simulink model "npc_controller"  (R2022a)
settings: Solver=FixedStepDiscrete  StartTime=0.0  StopTime=20  RelTol=1e-3  EnableMultiTasking=on
values from neighbouring files (symbols this model uses):
  Tsw = 1.5E-5    [param.sldd]
undefined symbols (not defined in the file or in its folder): CAN_O_INT, CANA_BASE, Down, GPTRIP1SEL, GPTRIP2SEL, GPTRIP3SEL, TZ1, TZ2, TZ3, Up
libraries: simulink x153, hdlsllib x90, c2802xlib x34, c2837xDlib x18, c280xlib x12, canmsglib x9, c2838xlib x8, idelinklib_common x3, c2806xlib x2, slpidlib x2, c28004xlib x2, c281xlib x2
(part 42 of 45)

== system npc_controller/IDLE_AND_TIMER/codegen/CAN_Task/Tx_Handler/Run Tx Routine/TxStatusData/Tx Pri3 ID132/Float Data to Bytes3 ==
  Float Data : Inport
  Resol. : Inport  Port=2
  Bit Shift : hdlsllib/Logic and Bit Operations/Bit Shift  mode=Shift Right Logical  N=8
  Bitwise AND : simulink/Logic and Bit Operations/Bitwise Operator  logicop=AND  UseBitMask=on  BitMask=bin2dec('0000000011111111')  BitMaskRealWorld=Stored Integer
  Bitwise AND1 : simulink/Logic and Bit Operations/Bitwise Operator  logicop=AND  UseBitMask=on  BitMask=hex2dec('FF00')  BitMaskRealWorld=Stored Integer
  Data Type Conversion : DataTypeConversion  OutDataTypeStr=uint8  SaturateOnIntegerOverflow=off  RndMeth=Floor
  Data Type Conversion1 : DataTypeConversion  OutDataTypeStr=uint8  SaturateOnIntegerOverflow=off  RndMeth=Floor
  Data Type Conversion2 : DataTypeConversion  OutDataTypeStr=uint16  SaturateOnIntegerOverflow=off  RndMeth=Floor
  Divide : Product  Inputs=*/
  u8Lsb : Outport
  u8Msb : Outport  Port=2
  wires:
  Data Type Conversion/1 -> u8Lsb/1
  Bitwise AND1/1 -> Bit Shift/1
  Data Type Conversion1/1 -> u8Msb/1
  Bitwise AND/1 -> Data Type Conversion/1
  Bit Shift/1 -> Data Type Conversion1/1
  Data Type Conversion2/1 -> Bitwise AND1/1, Bitwise AND/1  "u16toBytes_1"
  Divide/1 -> Data Type Conversion2/1
  Float Data/1 -> Divide/1
  Resol./1 -> Divide/2

== stateflow chart npc_controller/IDLE_AND_TIMER/codegen/Chart1 ==
  state INIT
    en:
    sim_control;
  (default) -> INIT
  INIT -> INIT
  events: sim_control output FUNCTION_CALL_EVENT

== stateflow chart npc_controller/CONTROL/STATE-MACHINE/CPU_CONTROL_200_Vpk ==
  state configGrid(grid_config,   sinlgeph_config) [function] [commented out]
  state enDigCmpMode [function]
  state configFutEn [function]
  state disDigCmpMode [function]
  state configFutDis [function]
  state theta = updatePll3p(van, vbn, vcn) [function] [commented out]
  state calib_ok = updateCalib(cnt_calib, van, vbn, vcn, ia, ib, ic) [function]
  state disablePwm [function]
  state tfv_v_UvpOvp = detectUvpOvp(Vpk) [function]
  state phx_en = detectZCPhA(vxn) [function]
  state phx_en = detectZCPhB(vxn) [function]
  state phx_en = detectZCPhC(vxn) [function]
  state vx_seq = updateSequencePhA(vxn, ix) [function]
  state vx_seq = updateSequencePhB(vxn, ix) [function]
  state vx_seq = updateSequencePhC(vxn, ix) [function]
  (default) -> (junction 597)
  (junction 598) -> (junction 531) [order 1] : [calib_ok]
  (junction 597) -> (junction 598) [order 1] : [start_cnt>33333] //50cycles
  (junction 531) -> (junction 14)
  (junction 597) -> (junction 601) [order 2] : {start_cnt++;}
  (junction 598) -> (junction 539) [order 2] : {
      | calib_ok = updateCalib(cnt_calib, van, vbn, vcn, ia, ib, ic);
      | state = 0;
      | }
  (junction 14) -> (junction 542) [order 2]
  (junction 14) -> (junction 128) [order 1] : [tfv_va || tfv_vb || tfv_vc || tfv_iphasea || tfv_iphaseb || tfv_iphasec || tfv_vbulk || tfv_vmid /*|| tfv_vtop*/ || tfv_vaux || tz_ocp || tz_ovp || fault]
      | {
      | fault = true;
      | state = 1;
      | }
  (junction 542) -> (junction 501)
  (junction 501) -> (junction 544) [order 2]
  (junction 501) -> (junction 490) [order 1] : [fut_en_req]
  (junction 544) -> (junction 504)
  (junction 490) -> (junction 492) [order 1] : [!fut_en]
  (junction 504) -> (junction 506) [order 1] : [fut_en]
  (junction 492) -> (junction 498) : {
      | configFutEn();
      | fut_en = true;
      | }
  (junction 490) -> (junction 494) [order 2]
  (junction 504) -> (junction 512) [order 2]
  (junction 506) -> (junction 508) : {
      | configFutDis();
      | fut_en = false;
      | }
  (junction 494) -> (junction 498)
  (junction 508) -> (junction 512)
  (junction 498) -> (junction 520) : {state = 2;}
  (junction 512) -> (junction 346)
  (junction 346) -> (junction 339) [order 1] : [vbulk > 618] //140V
  (junction 346) -> (junction 557) [order 2]
  (junction 339) -> (junction 329) : {
      | control_en = true;
      | enDigCmpMode();
      | }
  (junction 557) -> (junction 560) [order 1] : [vbulk < 530] //120V
  (junction 557) -> (junction 558) [order 2]
  (junction 560) -> (junction 559) : {control_en = false;}
  (junction 558) -> (junction 559)
  (junction 559) -> (junction 329)
  (junction 329) -> (junction 114) [order 1] : [control_en]
  (junction 114) -> (junction 266) [order 1] : [vbulk > 1104] //250V
  (junction 329) -> (junction 580) [order 2]
  (junction 114) -> (junction 263) [order 2]
  (junction 266) -> (junction 273) : {
      | eoss = false;
      | burst_en = true;
      | }
  (junction 263) -> (junction 264) [order 1] : [vbulk < 883] //200V
  (junction 263) -> (junction 267) [order 2]
  (junction 264) -> (junction 270) : {burst_en = false;}
  (junction 267) -> (junction 270)
  (junction 270) -> (junction 273)
  (junction 273) -> (junction 276) [order 1] : [burst_en]
  (junction 273) -> (junction 254) [order 2]
  (junction 276) -> (junction 327) : {
      | disablePwm();
      | va_seq = uint8(0); //forced zero
      | vb_seq = uint8(0);
      | vc_seq = uint8(0);
      | pha_en = false;
      | phb_en = false;
      | phc_en = false;
      | state = 5;
      | }
  (junction 254) -> (junction 606) [order 1] : [eoss]
      | //{tfv_v_UvpOvp = detectUvpOvp(Vpk)}
  (junction 606) -> (junction 256) [order 1] : [1/*!tfv_v_UvpOvp*/]
  (junction 254) -> (junction 97) [order 2]
  (junction 606) -> (junction 607) [order 2]
  (junction 256) -> (junction 101)
  (junction 580) -> (junction 581) [commented out] : [(grid_config_req != grid_config) || (singleph_config_req != singleph_config)]
  (junction 97) -> (junction 93) [order 1] : [(single(883)-vbulk) > single(50)] //11V ripple
  (junction 580) -> (junction 583)
  (junction 581) -> (junction 582) [commented out] : {
      | configGrid(grid_config,   singleph_config);
      | grid_config = grid_config_req;
      | singleph_config = singleph_config_req;
      | }
  (junction 97) -> (junction 110) [order 2]
  (junction 93) -> (junction 109) : {ref = vbulk + single(50);
      | eoss = false;}
  (junction 110) -> (junction 96) [order 1] : [(single(883)-vbulk) < single(-50)]
  (junction 110) -> (junction 94) [order 2] : {ref = single(883); //200V
      | eoss = true;}
  (junction 96) -> (junction 108) : {ref = vbulk - single(50);
      | eoss = false;}
  (junction 101) -> (junction 352) [order 1] : [pha_en]
  (junction 109) -> (junction 101)
  (junction 582) -> (junction 583) [commented out]
  (junction 94) -> (junction 108)
  (junction 108) -> (junction 109)
  (junction 101) -> (junction 356) [order 2] : {
      | va_seq = uint8(0);
      | pha_en = detectZCPhA(van);
      | }
  (junction 352) -> (junction 354) : {va_seq = updateSequencePhA(van, ia);}
  (junction 583) -> (junction 133)
  (junction 356) -> (junction 354)
  (junction 354) -> (junction 362) [order 1] : [phb_en]
  (junction 354) -> (junction 365) [order 2] : {
      | vb_seq = uint8(0);
      | phb_en = detectZCPhB(vbn);
      | }
  (junction 362) -> (junction 366) : {vb_seq = updateSequencePhB(vbn, ib);}
  (junction 365) -> (junction 366)
  (junction 366) -> (junction 367) [order 1] : [phc_en]
  (junction 366) -> (junction 370) [order 2] : {
      | vc_seq = uint8(0);
      | phc_en = detectZCPhC(vcn);
      | }
  (junction 367) -> (junction 372) : {vc_seq = updateSequencePhC(vcn, ic);}
  (junction 370) -> (junction 372)
  (junction 372) -> (junction 299) : {state = 4;}
  (junction 128) -> (junction 133) : //{calib_ok = false;} //calib_ok resets at fault or CAN command
  (junction 133) -> (junction 607)
  (junction 607) -> (junction 299) : {
      | disablePwm();
      | control_en = false;
      | eoss = false;
      | disDigCmpMode();
      | pha_en = false;
      | phb_en = false;
      | phc_en = false;
      | ref = vbulk;
      | state = 3;
      | }
  (junction 299) -> (junction 327)
  (junction 327) -> (junction 533)
  (junction 539) -> (junction 520)
  (junction 520) -> (junction 533)
  (junction 601) -> (junction 539)
  data: grid_config function_input double size=1; sinlgeph_config function_input double size=1; van function_input double size=1; vbn function_input double size=1; vcn function_input double size=1; theta function_output double size=1; calib_ok function_output; cnt_calib function_input uint16 size=1; van function_input single size=1; vbn function_input single size=1; vcn function_input single size=1; ia function_input single size=1; ib function_input single size=1; ic function_input single size=1; Vpk function_input; tfv_v_UvpOvp function_output; vxn function_input; phx_en function_output; vxn function_input; phx_en function_output; vxn function_input; phx_en function_output; vxn function_input; vx_seq function_output; ix function_input; vxn function_input; vx_seq function_output; ix function_input; vxn function_input; vx_seq function_output; ix function_input; state output uint16 =0; calib_ok output boolean =false; van input single; vbn input single; vcn input single; ia input single; ib input single; ic input single; tfv_vbulk data_store_memory; tfv_va data_store_memory; tfv_vmid data_store_memory; tfv_vb data_store_memory; tfv_vc data_store_memory; tfv_iphasea data_store_memory; tfv_iphaseb data_store_memory; tfv_iphasec data_store_memory; tfv_vtop data_store_memory; control_en output boolean =false; burst_en output boolean =false; eoss output boolean =false; ref output single =0; va_seq output uint8 =false; vb_seq output uint8 =false; vc_seq output uint8 =false; vbulk input single; fault local boolean =false; cnt_calib data_store_memory =0; theta data_store_memory =0; fut_en_req input uint8; fut_en local boolean =false; tfv_vaux data_store_memory; tz_ocp data_store_memory; tz_ovp data_store_memory; cnt_200ms local uint16 =0; pha_en output boolean =false; phb_en output boolean =false; phc_en output boolean =false; grid_config_req input uint8; singleph_config_req input uint8; grid_config local uint8 =0; singleph_config local uint8 =0; start_cnt local double; Vpk input single; tfv_v_UvpOvp local boolean

== stateflow chart npc_controller/CONTROL/STATE-MACHINE/CPU_CONTROL_750_Vpk ==
  state configGrid(grid_config,   sinlgeph_config) [function] [commented out]
  state enDigCmpMode [function]
  state configFutEn [function]
  state disDigCmpMode [function]
  state configFutDis [function]
  state theta = updatePll3p(van, vbn, vcn) [function] [commented out]
  state calib_ok = updateCalib(cnt_calib, van, vbn, vcn, ia, ib, ic) [function]
  state disablePwm [function]
  state tfv_v_UvpOvp = detectUvpOvp(Vpk) [function]
  state phx_en = detectZCPhA(vxn) [function]
  state phx_en = detectZCPhB(vxn) [function]
  state phx_en = detectZCPhC(vxn) [function]
  state vx_seq = updateSequencePhA(vxn, ix) [function]
  state vx_seq = updateSequencePhB(vxn, ix) [function]
  state vx_seq = updateSequencePhC(vxn, ix) [function]
  (default) -> (junction 597)
  (junction 598) -> (junction 531) [order 1] : [calib_ok]
  (junction 597) -> (junction 598) [order 1] : [start_cnt>33333] //50cycles
  (junction 531) -> (junction 14)
  (junction 597) -> (junction 601) [order 2] : {start_cnt++;}
  (junction 598) -> (junction 539) [order 2] : {
      | calib_ok = updateCalib(cnt_calib, van, vbn, vcn, ia, ib, ic);
      | state = 0;
      | }
  (junction 14) -> (junction 542) [order 2]
  (junction 14) -> (junction 128) [order 1] : [tfv_va || tfv_vb || tfv_vc || tfv_iphasea || tfv_iphaseb || tfv_iphasec || tfv_vbulk || tfv_vmid /*|| tfv_vtop*/ || tfv_vaux || tz_ocp || tz_ovp || fault]
      | {
      | fault = true;
      | state = 1;
      | }
  (junction 542) -> (junction 501)
  (junction 501) -> (junction 544) [order 2]
  (junction 501) -> (junction 490) [order 1] : [fut_en_req]
  (junction 544) -> (junction 504)
  (junction 490) -> (junction 492) [order 1] : [!fut_en]
  (junction 504) -> (junction 506) [order 1] : [fut_en]
  (junction 492) -> (junction 498) : {
      | configFutEn();
      | fut_en = true;
      | }
  (junction 490) -> (junction 494) [order 2]
  (junction 504) -> (junction 512) [order 2]
  (junction 506) -> (junction 508) : {
      | configFutDis();
      | fut_en = false;
      | }
  (junction 494) -> (junction 498)
  (junction 508) -> (junction 512)
  (junction 498) -> (junction 520) : {state = 2;}
  (junction 512) -> (junction 346)
  (junction 346) -> (junction 339) [order 1] : [vbulk > 2872] //650V
  (junction 346) -> (junction 557) [order 2]
  (junction 339) -> (junction 329) : {
      | control_en = true;
      | enDigCmpMode();
      | }
  (junction 557) -> (junction 560) [order 1] : [vbulk < 2430] //550V
  (junction 557) -> (junction 558) [order 2]
  (junction 560) -> (junction 559) : {control_en = false;}
  (junction 558) -> (junction 559)
  (junction 559) -> (junction 329)
  (junction 329) -> (junction 114) [order 1] : [control_en]
  (junction 114) -> (junction 266) [order 1] : [vbulk > 3711] //840V
  (junction 329) -> (junction 580) [order 2]
  (junction 114) -> (junction 263) [order 2]
  (junction 266) -> (junction 273) : {
      | eoss = false;
      | burst_en = true;
      | }
  (junction 263) -> (junction 264) [order 1] : [vbulk < 3313] //750V
  (junction 263) -> (junction 267) [order 2]
  (junction 264) -> (junction 270) : {burst_en = false;}
  (junction 267) -> (junction 270)
  (junction 270) -> (junction 273)
  (junction 273) -> (junction 276) [order 1] : [burst_en]
  (junction 273) -> (junction 254) [order 2]
  (junction 276) -> (junction 327) : {
      | disablePwm();
      | va_seq = uint8(0); //forced zero
      | vb_seq = uint8(0);
      | vc_seq = uint8(0);
      | pha_en = false;
      | phb_en = false;
      | phc_en = false;
      | state = 5;
      | }
  (junction 254) -> (junction 606) [order 1] : [eoss]
      | //{tfv_v_UvpOvp = detectUvpOvp(Vpk)}
  (junction 606) -> (junction 256) [order 1] : [1/*!tfv_v_UvpOvp*/]
  (junction 254) -> (junction 97) [order 2]
  (junction 606) -> (junction 607) [order 2]
  (junction 256) -> (junction 101)
  (junction 580) -> (junction 581) [commented out] : [(grid_config_req != grid_config) || (singleph_config_req != singleph_config)]
  (junction 97) -> (junction 93) [order 1] : [(single(3313)-vbulk) > single(50)] //11V ripple
  (junction 580) -> (junction 583)
  (junction 581) -> (junction 582) [commented out] : {
      | configGrid(grid_config,   singleph_config);
      | grid_config = grid_config_req;
      | singleph_config = singleph_config_req;
      | }
  (junction 97) -> (junction 110) [order 2]
  (junction 93) -> (junction 109) : {ref = vbulk + single(50);
      | eoss = false;}
  (junction 110) -> (junction 96) [order 1] : [(single(3313)-vbulk) < single(-50)]
  (junction 110) -> (junction 94) [order 2] : {ref = single(3313); //750V
      | eoss = true;}
  (junction 96) -> (junction 108) : {ref = vbulk - single(50);
      | eoss = false;}
  (junction 101) -> (junction 352) [order 1] : [pha_en]
  (junction 109) -> (junction 101)
  (junction 582) -> (junction 583) [commented out]
  (junction 94) -> (junction 108)
  (junction 108) -> (junction 109)
  (junction 101) -> (junction 356) [order 2] : {
      | va_seq = uint8(0);
      | pha_en = detectZCPhA(van);
      | }
  (junction 352) -> (junction 354) : {va_seq = updateSequencePhA(van, ia);}
  (junction 583) -> (junction 133)
  (junction 356) -> (junction 354)
  (junction 354) -> (junction 362) [order 1] : [phb_en]
  (junction 354) -> (junction 365) [order 2] : {
      | vb_seq = uint8(0);
      | phb_en = detectZCPhB(vbn);
      | }
  (junction 362) -> (junction 366) : {vb_seq = updateSequencePhB(vbn, ib);}
  (junction 365) -> (junction 366)
  (junction 366) -> (junction 367) [order 1] : [phc_en]
  (junction 366) -> (junction 370) [order 2] : {
      | vc_seq = uint8(0);
      | phc_en = detectZCPhC(vcn);
      | }
  (junction 367) -> (junction 372) : {vc_seq = updateSequencePhC(vcn, ic);}
  (junction 370) -> (junction 372)
  (junction 372) -> (junction 299) : {state = 4;}
  (junction 128) -> (junction 133) : //{calib_ok = false;} //calib_ok resets at fault or CAN command
  (junction 133) -> (junction 607)
  (junction 607) -> (junction 299) : {
      | disablePwm();
      | control_en = false;
      | eoss = false;
      | disDigCmpMode();
      | pha_en = false;
      | phb_en = false;
      | phc_en = false;
      | ref = vbulk;
      | state = 3;
      | }
  (junction 299) -> (junction 327)
  (junction 327) -> (junction 533)
  (junction 539) -> (junction 520)
  (junction 520) -> (junction 533)
  (junction 601) -> (junction 539)
  data: grid_config function_input double size=1; sinlgeph_config function_input double size=1; van function_input double size=1; vbn function_input double size=1; vcn function_input double size=1; theta function_output double size=1; calib_ok function_output; cnt_calib function_input uint16 size=1; van function_input single size=1; vbn function_input single size=1; vcn function_input single size=1; ia function_input single size=1; ib function_input single size=1; ic function_input single size=1; Vpk function_input; tfv_v_UvpOvp function_output; vxn function_input; phx_en function_output; vxn function_input; phx_en function_output; vxn function_input; phx_en function_output; vxn function_input; vx_seq function_output; ix function_input; vxn function_input; vx_seq function_output; ix function_input; vxn function_input; vx_seq function_output; ix function_input; state output uint16 =0; calib_ok output boolean =false; van input single; vbn input single; vcn input single; ia input single; ib input single; ic input single; tfv_vbulk data_store_memory; tfv_va data_store_memory; tfv_vmid data_store_memory; tfv_vb data_store_memory; tfv_vc data_store_memory; tfv_iphasea data_store_memory; tfv_iphaseb data_store_memory; tfv_iphasec data_store_memory; tfv_vtop data_store_memory; control_en output boolean =false; burst_en output boolean =false; eoss output boolean =false; ref output single =0; va_seq output uint8 =false; vb_seq output uint8 =false; vc_seq output uint8 =false; vbulk input single; fault local boolean =false; cnt_calib data_store_memory =0; theta data_store_memory =0; fut_en_req input uint8; fut_en local boolean =false; tfv_vaux data_store_memory; tz_ocp data_store_memory; tz_ovp data_store_memory; cnt_200ms local uint16 =0; pha_en output boolean =false; phb_en output boolean =false; phc_en output boolean =false; grid_config_req input uint8; singleph_config_req input uint8; grid_config local uint8 =0; singleph_config local uint8 =0; start_cnt local double; Vpk input single; tfv_v_UvpOvp local boolean

== stateflow chart npc_controller/CONTROL/STATE-MACHINE/CPU_CONTROL_750_A2_precharge_pfc_ok1 ==
  state configGrid(grid_config,   sinlgeph_config) [function] [commented out]
  state enDigCmpMode [function]
  state configFutEn [function]
  state disDigCmpMode [function]
  state configFutDis [function]
  state theta = updatePll3p(van, vbn, vcn) [function] [commented out]
  state calib_ok = updateCalib(cnt_calib, van, vbn, vcn, ia, ib, ic) [function]
  state disablePwm [function]
  state tfv_v_UvpOvp = detectUvpOvp(Vpk) [function]
  state tfv_v_UvpOvp = detectUvpOvp1(Vpk) [function] [commented out]
  state phx_en = detectZCPhA(vxn) [function]
  state phx_en = detectZCPhB(vxn) [function]
  state phx_en = detectZCPhC(vxn) [function]
  state vx_seq = updateSequencePhA(vxn, ix) [function]
  state vx_seq = updateSequencePhB(vxn, ix) [function]
  state vx_seq = updateSequencePhC(vxn, ix) [function]
  (default) -> (junction 597)
  (junction 598) -> (junction 531) [order 1] : [calib_ok]
      | {tfv_v_UvpOvp = detectUvpOvp(Vpk)}
  (junction 597) -> (junction 598) [order 1] : [start_cnt>33333] //50cycles
  (junction 531) -> (junction 14)
  (junction 597) -> (junction 601) [order 2] : {start_cnt++;}
      | //exit
  (junction 598) -> (junction 539) [order 2] : {
      | calib_ok = updateCalib(cnt_calib, van, vbn, vcn, ia, ib, ic);
      | state = 0;
      | }
      | //exit
  (junction 14) -> (junction 542) [order 2]
  (junction 542) -> (junction 504) [order 2]
  (junction 504) -> (junction 506) [order 1] : [fut_en]
  (junction 14) -> (junction 128) [order 1] : /*fault latch*/
      | [tfv_va || tfv_vb || tfv_vc || tfv_iphasea || tfv_iphaseb || tfv_iphasec || tfv_vbulk || tfv_vmid /*|| tfv_vtop*/ || tfv_vaux || tz_ocp || tz_ovp || fault]
      | {
      | fault = true;
      | state = 1;
      | }//
      | //turn OFF
  (junction 542) -> (junction 501) [order 1]
  (junction 504) -> (junction 512) [order 2]
  (junction 506) -> (junction 508) : {
      | configFutDis();
      | fut_en = false;
      | }
  (junction 508) -> (junction 512)
  (junction 501) -> (junction 490) : [fut_en_req]
  (junction 512) -> (junction 739)
  (junction 739) -> (junction 742) [commented out]
  (junction 490) -> (junction 492) [order 1] : [!fut_en]
  (junction 739) -> (junction 745) [order 2]
  (junction 742) -> (junction 735) [commented out] : [control_en]
  (junction 492) -> (junction 498) : {
      | configFutEn();
      | fut_en = true;
      | }
  (junction 490) -> (junction 494) [order 2]
  (junction 745) -> (junction 762) : //turn OFF
  (junction 739) -> (junction 734) [order 1] : [!tfv_v_UvpOvp]//check ac_ok at start
  (junction 494) -> (junction 498)
  (junction 735) -> (junction 734) [commented out]
  (junction 498) -> (junction 520) : {state = 2;}
  (junction 734) -> (junction 721)
  (junction 676) -> (junction 679) [order 1] : [control_en]
  (junction 721) -> (junction 712) [order 1] : [!pfc_en]
      | {state = 6;}
      | //turn OFF
      | //relay OFF
  (junction 721) -> (junction 676) [order 2]
  (junction 679) -> (junction 678)
  (junction 712) -> (junction 713)
  (junction 676) -> (junction 346) [order 2]
  (junction 346) -> (junction 626) [order 1] : [abs(1.9797*2*Vpk-vbulk) < 50]
  (junction 346) -> (junction 558) [order 2]
  (junction 626) -> (junction 658) : {relay_ctrl = 1; //pre-charge relay ON
      | }
  (junction 658) -> (junction 678)
  (junction 678) -> (junction 622) [order 1] : [relay_ctrl]
  (junction 558) -> (junction 658)
  (junction 622) -> (junction 624) [order 1] : [relay_cnt > 3300] //PWM ON with 40ms delay
  (junction 624) -> (junction 754) [order 1] : [control_en]
  (junction 678) -> (junction 707) [order 2] : //exit
  (junction 622) -> (junction 623) [order 2] : {relay_cnt++;}
      | //exit
  (junction 624) -> (junction 699) [order 2]
  (junction 754) -> (junction 684)
  (junction 699) -> (junction 698) [order 1] : [vbulk > 2872]
      | //140V(618),650V(2872)
  (junction 699) -> (junction 692) [order 2]
  (junction 698) -> (junction 696) : {
      | control_en = 1; //PWM ON
      | enDigCmpMode();
      | }
  (junction 692) -> (junction 689) [order 1] : [vbulk < 2430]
      | //120V(530),550V(2430)
  (junction 692) -> (junction 691) [order 2]
  (junction 689) -> (junction 695) : {
      | control_en = false;
      | }
  (junction 684) -> (junction 114) [order 1] : [control_en]
  (junction 114) -> (junction 266) [order 1] : [vbulk > 3711]
      | //250V(1104),840V(3711)
  (junction 696) -> (junction 684)
  (junction 691) -> (junction 695)
  (junction 695) -> (junction 696)
  (junction 684) -> (junction 665) [order 2] : //exit
  (junction 114) -> (junction 263) [order 2]
  (junction 266) -> (junction 273) : {
      | eoss = false;
      | burst_en = true;
      | }
  (junction 263) -> (junction 264) [order 1] : [vbulk < 3313]
      | //200V(883),750V(3313)
  (junction 263) -> (junction 267) [order 2]
  (junction 264) -> (junction 270) : {burst_en = false;}
  (junction 267) -> (junction 270)
  (junction 270) -> (junction 273)
  (junction 273) -> (junction 276) [order 1] : [burst_en]
  (junction 273) -> (junction 254) [order 2]
  (junction 276) -> (junction 327) : {
      | disablePwm();
      | va_seq = uint8(0); //forced zero
      | vb_seq = uint8(0);
      | vc_seq = uint8(0);
      | pha_en = false;
      | phb_en = false;
      | phc_en = false;
      | state = 5;
      | }
  (junction 254) -> (junction 606) [order 1] : [eoss]
      | //{tfv_v_UvpOvp = detectUvpOvp(Vpk)}
  (junction 606) -> (junction 256) [order 1] : [1/*!tfv_v_UvpOvp*/]
  (junction 256) -> (junction 648) [order 1] : [eoss_cnt > 6667]//5cycles delay after SS for PFC_OK
  (junction 254) -> (junction 97) [order 2]
  (junction 606) -> (junction 607) [order 2] : //turn OFF
  (junction 256) -> (junction 101) [order 2] : {
      | eoss_cnt++;
      | pfc_ok = 0;
      | }
  (junction 648) -> (junction 647) : {pfc_ok = 1;
      | /*eoss_cnt = 13100;*/}
  (junction 580) -> (junction 581) [commented out] : [(grid_config_req != grid_config) || (singleph_config_req != singleph_config)]
  (junction 97) -> (junction 93) [order 1] : [(single(3133)-vbulk) > single(10)] //2.2V ripple
  (junction 580) -> (junction 583) [commented out]
  (junction 581) -> (junction 582) [commented out] : {
      | configGrid(grid_config,   singleph_config);
      | grid_config = grid_config_req;
      | singleph_config = singleph_config_req;
      | }
  (junction 97) -> (junction 110) [order 2]
  (junction 93) -> (junction 109) : {ref = vbulk + single(1);
      | eoss = false;}
  (junction 110) -> (junction 96) [order 1] : [(single(3313)-vbulk) < single(-10)]
  (junction 110) -> (junction 94) [order 2] : {ref = single(3313);
      | //200V(883), 750V(3313)
      | eoss = true;}
  (junction 96) -> (junction 108) : {ref = vbulk - single(1);
      | eoss = false;}
  (junction 101) -> (junction 647)
  (junction 647) -> (junction 352) [order 1] : [pha_en]
  (junction 109) -> (junction 101)
  (junction 582) -> (junction 583) [commented out]
  (junction 94) -> (junction 108)
  (junction 108) -> (junction 109)
  (junction 647) -> (junction 356) [order 2] : {
      | va_seq = uint8(0);
      | pha_en = detectZCPhA(van);
      | }
  (junction 352) -> (junction 354) : {va_seq = updateSequencePhA(van, ia);}
  (junction 583) -> (junction 133) [commented out]
  (junction 356) -> (junction 354)
  (junction 354) -> (junction 362) [order 1] : [phb_en]
  (junction 354) -> (junction 365) [order 2] : {
      | vb_seq = uint8(0);
      | phb_en = detectZCPhB(vbn);
      | }
  (junction 362) -> (junction 366) : {vb_seq = updateSequencePhB(vbn, ib);}
  (junction 365) -> (junction 366)
  (junction 366) -> (junction 367) [order 1] : [phc_en]
  (junction 366) -> (junction 370) [order 2] : {
      | vc_seq = uint8(0);
      | phc_en = detectZCPhC(vcn);
      | }
  (junction 367) -> (junction 372) : {vc_seq = updateSequencePhC(vcn, ic);}
  (junction 370) -> (junction 372)
  (junction 372) -> (junction 299) : {state = 4;}
  (junction 133) -> (junction 607)
  (junction 757) -> (junction 635) [order 1] : [!pfc_en]
  (junction 635) -> (junction 299) [order 1] : [relayOff_cnt>2600] //40ms delay to turn-OFF pre-charge relay
      | {
      | relay_ctrl = 0; //pre-charge relay OFF
      | relayOff_cnt = 0;
      | relay_cnt = 0;
      | eoss_cnt = 0;
      | }
  (junction 128) -> (junction 762) : //{calib_ok = false;} //calib_ok resets at fault or CAN command
  (junction 762) -> (junction 713)
  (junction 713) -> (junction 133)
  (junction 299) -> (junction 327)
  (junction 607) -> (junction 757) : {
      | disablePwm();
      | //control_en = false;
      | eoss = false;
      | disDigCmpMode();
      | pha_en = false;
      | phb_en = false;
      | phc_en = false;
      | ref = vbulk;
      | state = 3;
      | pfc_ok = 0;
      | control_en = false;
      | }
  (junction 635) -> (junction 637) [order 2] : {relayOff_cnt++;}
  (junction 632) -> (junction 299)
  (junction 327) -> (junction 533)
  (junction 757) -> (junction 759) [order 2]
  (junction 637) -> (junction 632)
  (junction 539) -> (junction 520)
  (junction 520) -> (junction 731)
  (junction 731) -> (junction 707)
  (junction 707) -> (junction 623)
  (junction 623) -> (junction 665)
  (junction 665) -> (junction 759)
  (junction 759) -> (junction 533)
  (junction 601) -> (junction 539)
  data: grid_config function_input double size=1; sinlgeph_config function_input double size=1; van function_input double size=1; vbn function_input double size=1; vcn function_input double size=1; theta function_output double size=1; calib_ok function_output; cnt_calib function_input uint16 size=1; van function_input single size=1; vbn function_input single size=1; vcn function_input single size=1; ia function_input single size=1; ib function_input single size=1; ic function_input single size=1; Vpk function_input; tfv_v_UvpOvp function_output; Vpk function_input double size=1; tfv_v_UvpOvp function_output double size=1; vxn function_input; phx_en function_output; vxn function_input; phx_en function_output; vxn function_input; phx_en function_output; vxn function_input; vx_seq function_output; ix function_input; vxn function_input; vx_seq function_output; ix function_input; vxn function_input; vx_seq function_output; ix function_input; state output uint16 =0; calib_ok output boolean =false; van input single; vbn input single; vcn input single; ia input single; ib input single; ic input single; tfv_vbulk data_store_memory; tfv_va data_store_memory; tfv_vmid data_store_memory; tfv_vb data_store_memory; tfv_vc data_store_memory; tfv_iphasea data_store_memory; tfv_iphaseb data_store_memory; tfv_iphasec data_store_memory; tfv_vtop data_store_memory; control_en output boolean =false; burst_en output boolean =false; eoss output boolean =false; ref output single =0; va_seq output uint8 =false; vb_seq output uint8 =false; vc_seq output uint8 =false; vbulk input single; fault local boolean =false; cnt_calib data_store_memory =0; theta data_store_memory =0; fut_en_req input uint8; fut_en local boolean =false; tfv_vaux data_store_memory; tz_ocp data_store_memory; tz_ovp data_store_memory; cnt_200ms local uint16 =0; pha_en output boolean =false; phb_en output boolean =false; phc_en output boolean =false; grid_config_req input uint8; singleph_config_req input uint8; grid_config local uint8 =0; singleph_config local uint8 =0; start_cnt local double; Vpk input single; relayOff_cnt local double; relay_cnt local double; pfc_ok output boolean; eoss_cnt local double; relay_ctrl output boolean; pfc_en input; tfv_v_UvpOvp output boolean

== stateflow chart npc_controller/CONTROL/STATE-MACHINE/CPU_CONTROL_750_A2_precharge_pfc_ok1/detectUvpOvp/OVP ==
  (default) -> (junction 5)
  (junction 5) -> (junction 4) [order 1] : [Vpk1 > 773]
      | %65Vacrms(205),245Vrms(773)
  (junction 5) -> (junction 7) [order 2]
  (junction 4) -> (junction 6) : {
      | tfv_v_Ovp = 1; %set the OVP flag
      | }
  (junction 7) -> (junction 2) [order 1] : [Vpk1 < 741]
      | %54Vacrms(170),235Vrms(741)
  (junction 7) -> (junction 1) [order 2]
  (junction 2) -> (junction 3) : {
      | tfv_v_Ovp = 0;
      | }
  (junction 1) -> (junction 3)
  (junction 3) -> (junction 6)
  data: Vpk1 input single; tfv_v_Ovp output double

== matlab function npc_controller/CONTROL/CONTROL/false/CLA_CONTROL/CONTROL/MATLAB Function1 ==
  data: in input single; Vpeak output single
function Vpeak = SQRT(in)

%#codegen
Vpeak = single(0);
if isequal(coder.target,'rtw')  
    Vpeak = coder.ceval('CLAsqrt', in);
else
    Vpeak = sqrt(in);
end
end

% Vpeak = CLAsqrt(2/3*(va*va + vb*vb + vc*vc));
% 
% ua = va/Vpeak;
% 
% ub = vb/Vpeak;
% 
% uc = vc/Vpeak;
% 
% end


% function out = Div(num,den)
% 
% %#codegen
% out = single(0);
% if isequal(coder.target,'rtw')  
%     out = coder.ceval('CLAdiv', num, den);
% else
%     out = num/den;
% end
% end

== matlab function npc_controller/CONTROL/CONTROL/false/CLA_CONTROL/CONTROL/MATLAB Function2 ==
  data: va input single; out output single; vb input; vc input
function out = fcn(va, vb, vc)

out = 2/3*(va*va + vb*vb + vc*vc);

% ua = va/Vpeak;
% 
% ub = vb/Vpeak;
% 
% uc = vc/Vpeak;
% 
end


% function out = Div(num,den)
% 
% %#codegen
% out = single(0);
% if isequal(coder.target,'rtw')  
%     out = coder.ceval('CLAdiv', num, den);
% else
%     out = num/den;
% end
% end

== stateflow chart npc_controller/IDLE_AND_TIMER/codegen/TIMER_100MS/contstruct_can_msg/Chart ==
  (default) -> (junction 6)
  (junction 6) -> (junction 9) : {
      | can_msg[0] = uint8(func_id); //tmp_func_id;
      | can_msg[1] = uint8(data>>8);
      | can_msg[2] = uint8(data) ;
      | }
  data: func_id input uint16 size=1; data input uint16 size=1; can_msg output uint8 size=8 =[0 0 0 0 0 0 0 0]

== matlab function npc_controller/CONTROL/CONTROL/false/CLA_CONTROL/CONTROL/ubn ==
  data: num input; out output; den input
function out = Div(num,den)

%#codegen
out = single(0);
if isequal(coder.target,'rtw')  
    out = coder.ceval('CLAdiv', num, den);
else
    out = num/den;
end
end

== matlab function npc_controller/CONTROL/CONTROL/false/CLA_CONTROL/CONTROL/ucn ==
  data: num input; out output; den input
function out = Div(num,den)

%#codegen
out = single(0);
if isequal(coder.target,'rtw')  
    out = coder.ceval('CLAdiv', num, den);
else
    out = num/den;
end
end

== stateflow chart npc_controller/CONTROL/STATE-MACHINE/CPU_CONTROL_750_precharge_pfc_ok2 ==
  state configGrid(grid_config,   sinlgeph_config) [function] [commented out]
  state enDigCmpMode [function]
  state configFutEn [function]
  state disDigCmpMode [function]
  state configFutDis [function]
  state theta = updatePll3p(van, vbn, vcn) [function] [commented out]
  state calib_ok = updateCalib(cnt_calib, van, vbn, vcn, ia, ib, ic) [function]
  state disablePwm [function]
  state tfv_v_UvpOvp = detectUvpOvp(Vpk) [function]
  state tfv_v_UvpOvp = detectUvpOvp1(Vpk) [function] [commented out]
  state phx_en = detectZCPhA(vxn) [function]
  state phx_en = detectZCPhB(vxn) [function]
  state phx_en = detectZCPhC(vxn) [function]
  state vx_seq = updateSequencePhA(vxn, ix) [function]
  state vx_seq = updateSequencePhB(vxn, ix) [function]
  state vx_seq = updateSequencePhC(vxn, ix) [function]
  (default) -> (junction 597)
  (junction 598) -> (junction 531) [order 1] : [calib_ok]
      | {tfv_v_UvpOvp = detectUvpOvp(Vpk)}
  (junction 597) -> (junction 598) [order 1] : [start_cnt>33333] //50cycles
  (junction 531) -> (junction 14)
  (junction 597) -> (junction 601) [order 2] : {start_cnt++;}
      | //exit
  (junction 598) -> (junction 539) [order 2] : {
      | calib_ok = updateCalib(cnt_calib, van, vbn, vcn, ia, ib, ic);
      | state = 0;
      | }
      | //exit
  (junction 14) -> (junction 542) [order 2]
  (junction 542) -> (junction 504) [order 2]
  (junction 504) -> (junction 506) [order 1] : [fut_en]
  (junction 14) -> (junction 128) [order 1] : /*fault latch*/
      | [tfv_va || tfv_vb || tfv_vc || tfv_iphasea || tfv_iphaseb || tfv_iphasec || tfv_vbulk || tfv_vmid /*|| tfv_vtop*/ || tfv_vaux || tz_ocp || tz_ovp || fault]
      | {
      | fault = true;
      | state = 1;
      | }//
      | //turn OFF
  (junction 542) -> (junction 501) [order 1]
  (junction 504) -> (junction 512) [order 2]
  (junction 506) -> (junction 508) : {
      | configFutDis();
      | fut_en = false;
      | }
  (junction 508) -> (junction 512)
  (junction 501) -> (junction 490) : [fut_en_req]
  (junction 512) -> (junction 739)
  (junction 739) -> (junction 742) [commented out]
  (junction 490) -> (junction 492) [order 1] : [!fut_en]
  (junction 739) -> (junction 745) [order 2]
  (junction 742) -> (junction 735) [commented out] : [control_en]
  (junction 492) -> (junction 498) : {
      | configFutEn();
      | fut_en = true;
      | }
  (junction 490) -> (junction 494) [order 2]
  (junction 745) -> (junction 762) : //turn OFF
  (junction 739) -> (junction 734) [order 1] : [!tfv_v_UvpOvp]//check ac_ok at start
  (junction 494) -> (junction 498)
  (junction 735) -> (junction 734) [commented out]
  (junction 498) -> (junction 520) : {state = 2;}
  (junction 734) -> (junction 721)
  (junction 676) -> (junction 679) [order 1] : [control_en]
  (junction 721) -> (junction 712) [order 1] : [!pfc_en]
      | {state = 6;}
      | //turn OFF
      | //relay OFF
  (junction 721) -> (junction 676) [order 2]
  (junction 679) -> (junction 678)
  (junction 712) -> (junction 713)
  (junction 676) -> (junction 346) [order 2]
  (junction 346) -> (junction 626) [order 1] : [abs(1.9797*2*Vpk-vbulk) < 50]
  (junction 346) -> (junction 558) [order 2]
  (junction 626) -> (junction 658) : {relay_ctrl = 1; //pre-charge relay ON
      | }
  (junction 658) -> (junction 678)
  (junction 678) -> (junction 622) [order 1] : [relay_ctrl]
  (junction 558) -> (junction 658)
  (junction 622) -> (junction 624) [order 1] : [relay_cnt > 3300] //PWM ON with 40ms delay
  (junction 624) -> (junction 754) [order 1] : [control_en]
  (junction 678) -> (junction 707) [order 2] : //exit
  (junction 622) -> (junction 623) [order 2] : {relay_cnt++;}
      | //exit
  (junction 624) -> (junction 699) [order 2]
  (junction 754) -> (junction 684)
  (junction 699) -> (junction 698) [order 1] : [vbulk > 2872] //650V
  (junction 699) -> (junction 692) [order 2]
  (junction 698) -> (junction 696) : {
      | control_en = 1; //PWM ON
      | enDigCmpMode();
      | }
  (junction 692) -> (junction 689) [order 1] : [vbulk < 2430] //550V
  (junction 692) -> (junction 691) [order 2]
  (junction 689) -> (junction 695) : {
      | control_en = false;
      | }
  (junction 684) -> (junction 114) [order 1] : [control_en]
  (junction 114) -> (junction 266) [order 1] : [vbulk > 3711] //840V
  (junction 696) -> (junction 684)
  (junction 691) -> (junction 695)
  (junction 695) -> (junction 696)
  (junction 684) -> (junction 665) [order 2] : //exit
  (junction 114) -> (junction 263) [order 2]
  (junction 266) -> (junction 273) : {
      | eoss = false;
      | burst_en = true;
      | }
  (junction 263) -> (junction 264) [order 1] : [vbulk < 3313] //750V
  (junction 263) -> (junction 267) [order 2]
  (junction 264) -> (junction 270) : {burst_en = false;}
  (junction 267) -> (junction 270)
  (junction 270) -> (junction 273)
  (junction 273) -> (junction 276) [order 1] : [burst_en]
  (junction 273) -> (junction 254) [order 2]
  (junction 276) -> (junction 327) : {
      | disablePwm();
      | va_seq = uint8(0); //forced zero
      | vb_seq = uint8(0);
      | vc_seq = uint8(0);
      | pha_en = false;
      | phb_en = false;
      | phc_en = false;
      | state = 5;
      | }
  (junction 254) -> (junction 606) [order 1] : [eoss]
      | //{tfv_v_UvpOvp = detectUvpOvp(Vpk)}
  (junction 606) -> (junction 256) [order 1] : [1/*!tfv_v_UvpOvp*/]
  (junction 256) -> (junction 648) [order 1] : [eoss_cnt > 6667]//5cycles delay after SS for PFC_OK
  (junction 254) -> (junction 97) [order 2]
  (junction 606) -> (junction 607) [order 2] : //turn OFF
  (junction 256) -> (junction 101) [order 2] : {
      | eoss_cnt++;
      | pfc_ok = 0;
      | }
  (junction 648) -> (junction 647) : {pfc_ok = 1;
      | /*eoss_cnt = 13100;*/}
  (junction 580) -> (junction 581) [commented out] : [(grid_config_req != grid_config) || (singleph_config_req != singleph_config)]
  (junction 97) -> (junction 93) [order 1] : [(single(3313)-vbulk) > single(50)] //11V ripple
  (junction 580) -> (junction 583) [commented out]
  (junction 581) -> (junction 582) [commented out] : {
      | configGrid(grid_config,   singleph_config);
      | grid_config = grid_config_req;
      | singleph_config = singleph_config_req;
      | }
  (junction 97) -> (junction 110) [order 2]
  (junction 93) -> (junction 109) : {ref = vbulk + single(50);
      | eoss = false;}
  (junction 110) -> (junction 96) [order 1] : [(single(3313)-vbulk) < single(-50)]
  (junction 110) -> (junction 94) [order 2] : {ref = single(3313); //750V
      | eoss = true;}
  (junction 96) -> (junction 108) : {ref = vbulk - single(50);
      | eoss = false;}
  (junction 101) -> (junction 647)
  (junction 647) -> (junction 352) [order 1] : [pha_en]
  (junction 109) -> (junction 101)
  (junction 582) -> (junction 583) [commented out]
  (junction 94) -> (junction 108)
  (junction 108) -> (junction 109)
  (junction 647) -> (junction 356) [order 2] : {
      | va_seq = uint8(0);
      | pha_en = detectZCPhA(van);
      | }
  (junction 352) -> (junction 354) : {va_seq = updateSequencePhA(van, ia);}
  (junction 583) -> (junction 133) [commented out]
  (junction 356) -> (junction 354)
  (junction 354) -> (junction 362) [order 1] : [phb_en]
  (junction 354) -> (junction 365) [order 2] : {
      | vb_seq = uint8(0);
      | phb_en = detectZCPhB(vbn);
      | }
  (junction 362) -> (junction 366) : {vb_seq = updateSequencePhB(vbn, ib);}
  (junction 365) -> (junction 366)
  (junction 366) -> (junction 367) [order 1] : [phc_en]
  (junction 366) -> (junction 370) [order 2] : {
      | vc_seq = uint8(0);
      | phc_en = detectZCPhC(vcn);
      | }
  (junction 367) -> (junction 372) : {vc_seq = updateSequencePhC(vcn, ic);}
  (junction 370) -> (junction 372)
  (junction 372) -> (junction 299) : {state = 4;}
  (junction 133) -> (junction 607)
  (junction 757) -> (junction 635) [order 1] : [!pfc_en]
  (junction 635) -> (junction 299) [order 1] : [relayOff_cnt>2600] //40ms delay to turn-OFF pre-charge relay
      | {
      | relay_ctrl = 0; //pre-charge relay OFF
      | relayOff_cnt = 0;
      | relay_cnt = 0;
      | }
  (junction 128) -> (junction 762) : //{calib_ok = false;} //calib_ok resets at fault or CAN command
  (junction 762) -> (junction 713)
  (junction 713) -> (junction 133)
  (junction 299) -> (junction 327)
  (junction 607) -> (junction 757) : {
      | disablePwm();
      | //control_en = false;
      | eoss = false;
      | disDigCmpMode();
      | pha_en = false;
      | phb_en = false;
      | phc_en = false;
      | ref = vbulk;
      | state = 3;
      | pfc_ok = 0;
      | control_en = false;
      | eoss_cnt = 0;
      | }
  (junction 635) -> (junction 637) [order 2] : {relayOff_cnt++;}
  (junction 632) -> (junction 299)
  (junction 327) -> (junction 533)
  (junction 757) -> (junction 759) [order 2]
  (junction 637) -> (junction 632)
  (junction 539) -> (junction 520)
  (junction 520) -> (junction 731)
  (junction 731) -> (junction 707)
  (junction 707) -> (junction 623)
  (junction 623) -> (junction 665)
  (junction 665) -> (junction 759)
  (junction 759) -> (junction 533)
  (junction 601) -> (junction 539)
  data: grid_config function_input double size=1; sinlgeph_config function_input double size=1; van function_input double size=1; vbn function_input double size=1; vcn function_input double size=1; theta function_output double size=1; calib_ok function_output; cnt_calib function_input uint16 size=1; van function_input single size=1; vbn function_input single size=1; vcn function_input single size=1; ia function_input single size=1; ib function_input single size=1; ic function_input single size=1; Vpk function_input; tfv_v_UvpOvp function_output; Vpk function_input double size=1; tfv_v_UvpOvp function_output double size=1; vxn function_input; phx_en function_output; vxn function_input; phx_en function_output; vxn function_input; phx_en function_output; vxn function_input; vx_seq function_output; ix function_input; vxn function_input; vx_seq function_output; ix function_input; vxn function_input; vx_seq function_output; ix function_input; state output uint16 =0; calib_ok output boolean =false; van input single; vbn input single; vcn input single; ia input single; ib input single; ic input single; tfv_vbulk data_store_memory; tfv_va data_store_memory; tfv_vmid data_store_memory; tfv_vb data_store_memory; tfv_vc data_store_memory; tfv_iphasea data_store_memory; tfv_iphaseb data_store_memory; tfv_iphasec data_store_memory; tfv_vtop data_store_memory; control_en output boolean =false; burst_en output boolean =false; eoss output boolean =false; ref output single =0; va_seq output uint8 =false; vb_seq output uint8 =false; vc_seq output uint8 =false; vbulk input single; fault local boolean =false; cnt_calib data_store_memory =0; theta data_store_memory =0; fut_en_req input uint8; fut_en local boolean =false; tfv_vaux data_store_memory; tz_ocp data_store_memory; tz_ovp data_store_memory; cnt_200ms local uint16 =0; pha_en output boolean =false; phb_en output boolean =false; phc_en output boolean =false; grid_config_req input uint8; singleph_config_req input uint8; grid_config local uint8 =0; singleph_config local uint8 =0; start_cnt local double; Vpk input single; relayOff_cnt local double; relay_cnt local double; pfc_ok output boolean; eoss_cnt local double; relay_ctrl output boolean; pfc_en input; tfv_v_UvpOvp output boolean

== stateflow chart npc_controller/IDLE_AND_TIMER/codegen/TIMER_100MS/get_func_id_data/Chart2 ==
  (default) -> (junction 1)
  (junction 1) -> (junction 3) : {
      | va = uint16(adc.vbulk);
      | vb = uint16(adc.vb);
      | vc = uint16(adc.vc);
      | }
  data: adc local Bus: adc; va output uint16; vb output uint16; vc output uint16
